simulink model "fft_overlap_tomori"  (R2023b)
settings: Solver=VariableStepAuto  StartTime=0.0  StopTime=inf  RelTol=1e-3
InitFcn:
  | fftparrallelout
  | load('dataram.mat')
  | s= fi(exp(-1j*2*pi.*(0:63)/64),1,16,15);
  | fixed_point = fixdt(1,27,20);
  | fixed_pointu = fixdt(0,29,20);
  | fixed = fixdt(1,22,15);
  | const = fixdt(1,18,17);
  | addConst = fixdt(1,18,16);
  | f =10.4e6;
  | f1=45e6;
  | alpha1 =5;
  | beta1 = 0.00001 ;
  | beta2 = 0.99999 ;
  | beta3 = 23;
undefined symbols (not defined in the file or in its folder): j
libraries: dspxfrm3 x11, commrflib2 x4
(part 5 of 10)

== system fft_overlap_tomori/FFT64_outMuxed/64pointFFTchan/FFT64/complexmult23 ==
  x1 : Inport
  In3 : Inport  Port=2
  Add1 : Sum  OutDataTypeStr=addConst  RndMeth=Round
  Add2 : Sum  Inputs=+-  OutDataTypeStr=fixed  AccumDataTypeStr=fixed  RndMeth=Round
  Add20 : Sum  OutDataTypeStr=fixed  RndMeth=Round
  Add3 : Sum  Inputs=+-  OutDataTypeStr=fixed  AccumDataTypeStr=fixed  RndMeth=Round
  Add4 : Sum  Inputs=+-  OutDataTypeStr=fixed  AccumDataTypeStr=fixed  RndMeth=Round
  Complex to Real-Imag : ComplexToRealImag
  Complex to Real-Imag1 : ComplexToRealImag
  Constant : Constant  Commented=on  Value=1+j  OutDataTypeStr=fixdt(1,22, 15)  SampleTime=2e-8
  Constant1 : Constant  Commented=on  Value=1-j  OutDataTypeStr=fixdt(1,22, 15)  SampleTime=2e-8
  Data Type Conversion : DataTypeConversion  OutDataTypeStr=fixed  RndMeth=Round  SaturateOnIntegerOverflow=off
  Data Type Conversion1 : DataTypeConversion  OutDataTypeStr=fixed  RndMeth=Round  SaturateOnIntegerOverflow=off
  Data Type Conversion2 : DataTypeConversion  OutDataTypeStr=fixed  RndMeth=Round  SaturateOnIntegerOverflow=off
  Delay : Delay
  Delay1 : Delay
  Delay{3..14} (12 alike) : Delay  DelayLength=1
  Delay2 : Delay
  Display : Display  Commented=on
  Product : Product
  Product1 : Product
  Product2 : Product
  Real-Imag to Complex : RealImagToComplex
  Out1 : Outport
  wires:
  Delay14/1 -> Add4/2, Delay11/1
  Data Type Conversion2/1 -> Delay14/1
  Delay13/1 -> Add3/2, Add4/1
  Data Type Conversion1/1 -> Delay13/1
  Data Type Conversion/1 -> Delay12/1
  Delay12/1 -> Add3/1
  Add2/1 -> Real-Imag to Complex/2
  Delay11/1 -> Add2/2
  Delay10/1 -> Add2/1
  Delay9/1 -> Real-Imag to Complex/1
  Delay8/1 -> Product2/2
  Delay7/1 -> Product2/1
  Delay6/1 -> Product1/2
  Delay5/1 -> Product1/1
  Delay4/1 -> Product/2
  Delay3/1 -> Product/1
  Complex to Real-Imag1/2 -> Add1/2, Delay8/1
  Complex to Real-Imag/2 -> Add20/2, Delay7/1
  Complex to Real-Imag1/1 -> Add1/1, Delay6/1
  Complex to Real-Imag/1 -> Add20/1, Delay5/1
  Add1/1 -> Delay4/1
  Add20/1 -> Delay3/1
  Add3/1 -> Delay10/1
  Add4/1 -> Delay9/1
  Delay2/1 -> Data Type Conversion2/1
  Delay1/1 -> Data Type Conversion1/1
  Delay/1 -> Data Type Conversion/1
  Product2/1 -> Delay2/1
  Product1/1 -> Delay1/1
  Product/1 -> Delay/1
  x1/1 -> Complex to Real-Imag/1
  In3/1 -> Complex to Real-Imag1/1
  Real-Imag to Complex/1 -> Out1/1

== system fft_overlap_tomori/FFT64_outMuxed/64pointFFTchan/FFT64/complexmult24 ==
  x1 : Inport
  In3 : Inport  Port=2
  Add1 : Sum  OutDataTypeStr=addConst  RndMeth=Round
  Add2 : Sum  Inputs=+-  OutDataTypeStr=fixed  AccumDataTypeStr=fixed  RndMeth=Round
  Add20 : Sum  OutDataTypeStr=fixed  RndMeth=Round
  Add3 : Sum  Inputs=+-  OutDataTypeStr=fixed  AccumDataTypeStr=fixed  RndMeth=Round
  Add4 : Sum  Inputs=+-  OutDataTypeStr=fixed  AccumDataTypeStr=fixed  RndMeth=Round
  Complex to Real-Imag : ComplexToRealImag
  Complex to Real-Imag1 : ComplexToRealImag
  Constant : Constant  Commented=on  Value=1+j  OutDataTypeStr=fixdt(1,22, 15)  SampleTime=2e-8
  Constant1 : Constant  Commented=on  Value=1-j  OutDataTypeStr=fixdt(1,22, 15)  SampleTime=2e-8
  Data Type Conversion : DataTypeConversion  OutDataTypeStr=fixed  RndMeth=Round  SaturateOnIntegerOverflow=off
  Data Type Conversion1 : DataTypeConversion  OutDataTypeStr=fixed  RndMeth=Round  SaturateOnIntegerOverflow=off
  Data Type Conversion2 : DataTypeConversion  OutDataTypeStr=fixed  RndMeth=Round  SaturateOnIntegerOverflow=off
  Delay : Delay
  Delay1 : Delay
  Delay{3..14} (12 alike) : Delay  DelayLength=1
  Delay2 : Delay
  Display : Display  Commented=on
  Product : Product
  Product1 : Product
  Product2 : Product
  Real-Imag to Complex : RealImagToComplex
  Out1 : Outport
  wires:
  Real-Imag to Complex/1 -> Out1/1
  In3/1 -> Complex to Real-Imag1/1
  x1/1 -> Complex to Real-Imag/1
  Product/1 -> Delay/1
  Product1/1 -> Delay1/1
  Product2/1 -> Delay2/1
  Delay/1 -> Data Type Conversion/1
  Delay1/1 -> Data Type Conversion1/1
  Delay2/1 -> Data Type Conversion2/1
  Add4/1 -> Delay9/1
  Add3/1 -> Delay10/1
  Add20/1 -> Delay3/1
  Add1/1 -> Delay4/1
  Complex to Real-Imag/1 -> Delay5/1, Add20/1
  Complex to Real-Imag1/1 -> Delay6/1, Add1/1
  Complex to Real-Imag/2 -> Delay7/1, Add20/2
  Complex to Real-Imag1/2 -> Delay8/1, Add1/2
  Delay3/1 -> Product/1
  Delay4/1 -> Product/2
  Delay5/1 -> Product1/1
  Delay6/1 -> Product1/2
  Delay7/1 -> Product2/1
  Delay8/1 -> Product2/2
  Delay9/1 -> Real-Imag to Complex/1
  Delay10/1 -> Add2/1
  Delay11/1 -> Add2/2
  Add2/1 -> Real-Imag to Complex/2
  Delay12/1 -> Add3/1
  Data Type Conversion/1 -> Delay12/1
  Data Type Conversion1/1 -> Delay13/1
  Delay13/1 -> Add4/1, Add3/2
  Data Type Conversion2/1 -> Delay14/1
  Delay14/1 -> Delay11/1, Add4/2

== system fft_overlap_tomori/FFT64_outMuxed/64pointFFTchan/FFT64/complexmult25 ==
  x1 : Inport
  In3 : Inport  Port=2
  Add1 : Sum  OutDataTypeStr=addConst  RndMeth=Round
  Add2 : Sum  Inputs=+-  OutDataTypeStr=fixed  AccumDataTypeStr=fixed  RndMeth=Round
  Add20 : Sum  OutDataTypeStr=fixed  RndMeth=Round
  Add3 : Sum  Inputs=+-  OutDataTypeStr=fixed  AccumDataTypeStr=fixed  RndMeth=Round
  Add4 : Sum  Inputs=+-  OutDataTypeStr=fixed  AccumDataTypeStr=fixed  RndMeth=Round
  Complex to Real-Imag : ComplexToRealImag
  Complex to Real-Imag1 : ComplexToRealImag
  Constant : Constant  Commented=on  Value=1+j  OutDataTypeStr=fixdt(1,22, 15)  SampleTime=2e-8
  Constant1 : Constant  Commented=on  Value=1-j  OutDataTypeStr=fixdt(1,22, 15)  SampleTime=2e-8
  Data Type Conversion : DataTypeConversion  OutDataTypeStr=fixed  RndMeth=Round  SaturateOnIntegerOverflow=off
  Data Type Conversion1 : DataTypeConversion  OutDataTypeStr=fixed  RndMeth=Round  SaturateOnIntegerOverflow=off
  Data Type Conversion2 : DataTypeConversion  OutDataTypeStr=fixed  RndMeth=Round  SaturateOnIntegerOverflow=off
  Delay : Delay
  Delay1 : Delay
  Delay{3..14} (12 alike) : Delay  DelayLength=1
  Delay2 : Delay
  Display : Display  Commented=on
  Product : Product
  Product1 : Product
  Product2 : Product
  Real-Imag to Complex : RealImagToComplex
  Out1 : Outport
  wires:
  Delay14/1 -> Add4/2, Delay11/1
  Data Type Conversion2/1 -> Delay14/1
  Delay13/1 -> Add3/2, Add4/1
  Data Type Conversion1/1 -> Delay13/1
  Data Type Conversion/1 -> Delay12/1
  Delay12/1 -> Add3/1
  Add2/1 -> Real-Imag to Complex/2
  Delay11/1 -> Add2/2
  Delay10/1 -> Add2/1
  Delay9/1 -> Real-Imag to Complex/1
  Delay8/1 -> Product2/2
  Delay7/1 -> Product2/1
  Delay6/1 -> Product1/2
  Delay5/1 -> Product1/1
  Delay4/1 -> Product/2
  Delay3/1 -> Product/1
  Complex to Real-Imag1/2 -> Add1/2, Delay8/1
  Complex to Real-Imag/2 -> Add20/2, Delay7/1
  Complex to Real-Imag1/1 -> Add1/1, Delay6/1
  Complex to Real-Imag/1 -> Add20/1, Delay5/1
  Add1/1 -> Delay4/1
  Add20/1 -> Delay3/1
  Add3/1 -> Delay10/1
  Add4/1 -> Delay9/1
  Delay2/1 -> Data Type Conversion2/1
  Delay1/1 -> Data Type Conversion1/1
  Delay/1 -> Data Type Conversion/1
  Product2/1 -> Delay2/1
  Product1/1 -> Delay1/1
  Product/1 -> Delay/1
  x1/1 -> Complex to Real-Imag/1
  In3/1 -> Complex to Real-Imag1/1
  Real-Imag to Complex/1 -> Out1/1

== system fft_overlap_tomori/FFT64_outMuxed/64pointFFTchan/FFT64/complexmult26 ==
  x1 : Inport
  In3 : Inport  Port=2
  Add1 : Sum  OutDataTypeStr=addConst  RndMeth=Round
  Add2 : Sum  Inputs=+-  OutDataTypeStr=fixed  AccumDataTypeStr=fixed  RndMeth=Round
  Add20 : Sum  OutDataTypeStr=fixed  RndMeth=Round
  Add3 : Sum  Inputs=+-  OutDataTypeStr=fixed  AccumDataTypeStr=fixed  RndMeth=Round
  Add4 : Sum  Inputs=+-  OutDataTypeStr=fixed  AccumDataTypeStr=fixed  RndMeth=Round
  Complex to Real-Imag : ComplexToRealImag
  Complex to Real-Imag1 : ComplexToRealImag
  Constant : Constant  Commented=on  Value=1+j  OutDataTypeStr=fixdt(1,22, 15)  SampleTime=2e-8
  Constant1 : Constant  Commented=on  Value=1-j  OutDataTypeStr=fixdt(1,22, 15)  SampleTime=2e-8
  Data Type Conversion : DataTypeConversion  OutDataTypeStr=fixed  RndMeth=Round  SaturateOnIntegerOverflow=off
  Data Type Conversion1 : DataTypeConversion  OutDataTypeStr=fixed  RndMeth=Round  SaturateOnIntegerOverflow=off
  Data Type Conversion2 : DataTypeConversion  OutDataTypeStr=fixed  RndMeth=Round  SaturateOnIntegerOverflow=off
  Delay : Delay
  Delay1 : Delay
  Delay{3..14} (12 alike) : Delay  DelayLength=1
  Delay2 : Delay
  Display : Display  Commented=on
  Product : Product
  Product1 : Product
  Product2 : Product
  Real-Imag to Complex : RealImagToComplex
  Out1 : Outport
  wires:
  Real-Imag to Complex/1 -> Out1/1
  In3/1 -> Complex to Real-Imag1/1
  x1/1 -> Complex to Real-Imag/1
  Product/1 -> Delay/1
  Product1/1 -> Delay1/1
  Product2/1 -> Delay2/1
  Delay/1 -> Data Type Conversion/1
  Delay1/1 -> Data Type Conversion1/1
  Delay2/1 -> Data Type Conversion2/1
  Add4/1 -> Delay9/1
  Add3/1 -> Delay10/1
  Add20/1 -> Delay3/1
  Add1/1 -> Delay4/1
  Complex to Real-Imag/1 -> Delay5/1, Add20/1
  Complex to Real-Imag1/1 -> Delay6/1, Add1/1
  Complex to Real-Imag/2 -> Delay7/1, Add20/2
  Complex to Real-Imag1/2 -> Delay8/1, Add1/2
  Delay3/1 -> Product/1
  Delay4/1 -> Product/2
  Delay5/1 -> Product1/1
  Delay6/1 -> Product1/2
  Delay7/1 -> Product2/1
  Delay8/1 -> Product2/2
  Delay9/1 -> Real-Imag to Complex/1
  Delay10/1 -> Add2/1
  Delay11/1 -> Add2/2
  Add2/1 -> Real-Imag to Complex/2
  Delay12/1 -> Add3/1
  Data Type Conversion/1 -> Delay12/1
  Data Type Conversion1/1 -> Delay13/1
  Delay13/1 -> Add4/1, Add3/2
  Data Type Conversion2/1 -> Delay14/1
  Delay14/1 -> Delay11/1, Add4/2

== system fft_overlap_tomori/FFT64_outMuxed/64pointFFTchan/FFT64/complexmult27 ==
  x1 : Inport
  In3 : Inport  Port=2
  Add1 : Sum  OutDataTypeStr=addConst  RndMeth=Round
  Add2 : Sum  Inputs=+-  OutDataTypeStr=fixed  AccumDataTypeStr=fixed  RndMeth=Round
  Add20 : Sum  OutDataTypeStr=fixed  RndMeth=Round
  Add3 : Sum  Inputs=+-  OutDataTypeStr=fixed  AccumDataTypeStr=fixed  RndMeth=Round
  Add4 : Sum  Inputs=+-  OutDataTypeStr=fixed  AccumDataTypeStr=fixed  RndMeth=Round
  Complex to Real-Imag : ComplexToRealImag
  Complex to Real-Imag1 : ComplexToRealImag
  Constant : Constant  Commented=on  Value=1+j  OutDataTypeStr=fixdt(1,22, 15)  SampleTime=2e-8
  Constant1 : Constant  Commented=on  Value=1-j  OutDataTypeStr=fixdt(1,22, 15)  SampleTime=2e-8
  Data Type Conversion : DataTypeConversion  OutDataTypeStr=fixed  RndMeth=Round  SaturateOnIntegerOverflow=off
  Data Type Conversion1 : DataTypeConversion  OutDataTypeStr=fixed  RndMeth=Round  SaturateOnIntegerOverflow=off
  Data Type Conversion2 : DataTypeConversion  OutDataTypeStr=fixed  RndMeth=Round  SaturateOnIntegerOverflow=off
  Delay : Delay
  Delay1 : Delay
  Delay{3..14} (12 alike) : Delay  DelayLength=1
  Delay2 : Delay
  Display : Display  Commented=on
  Product : Product
  Product1 : Product
  Product2 : Product
  Real-Imag to Complex : RealImagToComplex
  Out1 : Outport
  wires:
  Delay14/1 -> Add4/2, Delay11/1
  Data Type Conversion2/1 -> Delay14/1
  Delay13/1 -> Add3/2, Add4/1
  Data Type Conversion1/1 -> Delay13/1
  Data Type Conversion/1 -> Delay12/1
  Delay12/1 -> Add3/1
  Add2/1 -> Real-Imag to Complex/2
  Delay11/1 -> Add2/2
  Delay10/1 -> Add2/1
  Delay9/1 -> Real-Imag to Complex/1
  Delay8/1 -> Product2/2
  Delay7/1 -> Product2/1
  Delay6/1 -> Product1/2
  Delay5/1 -> Product1/1
  Delay4/1 -> Product/2
  Delay3/1 -> Product/1
  Complex to Real-Imag1/2 -> Add1/2, Delay8/1
  Complex to Real-Imag/2 -> Add20/2, Delay7/1
  Complex to Real-Imag1/1 -> Add1/1, Delay6/1
  Complex to Real-Imag/1 -> Add20/1, Delay5/1
  Add1/1 -> Delay4/1
  Add20/1 -> Delay3/1
  Add3/1 -> Delay10/1
  Add4/1 -> Delay9/1
  Delay2/1 -> Data Type Conversion2/1
  Delay1/1 -> Data Type Conversion1/1
  Delay/1 -> Data Type Conversion/1
  Product2/1 -> Delay2/1
  Product1/1 -> Delay1/1
  Product/1 -> Delay/1
  x1/1 -> Complex to Real-Imag/1
  In3/1 -> Complex to Real-Imag1/1
  Real-Imag to Complex/1 -> Out1/1

== system fft_overlap_tomori/FFT64_outMuxed/64pointFFTchan/FFT64/complexmult3 ==
  x1 : Inport
  In3 : Inport  Port=2
  Add1 : Sum  OutDataTypeStr=addConst  RndMeth=Round
  Add2 : Sum  Inputs=+-  OutDataTypeStr=fixed  AccumDataTypeStr=fixed  RndMeth=Round
  Add20 : Sum  OutDataTypeStr=fixed  RndMeth=Round
  Add3 : Sum  Inputs=+-  OutDataTypeStr=fixed  AccumDataTypeStr=fixed  RndMeth=Round
  Add4 : Sum  Inputs=+-  OutDataTypeStr=fixed  AccumDataTypeStr=fixed  RndMeth=Round
  Complex to Real-Imag : ComplexToRealImag
  Complex to Real-Imag1 : ComplexToRealImag
  Constant : Constant  Commented=on  Value=1+j  OutDataTypeStr=fixdt(1,22, 15)  SampleTime=2e-8
  Constant1 : Constant  Commented=on  Value=1-j  OutDataTypeStr=fixdt(1,22, 15)  SampleTime=2e-8
  Data Type Conversion : DataTypeConversion  OutDataTypeStr=fixed  RndMeth=Round  SaturateOnIntegerOverflow=off
  Data Type Conversion1 : DataTypeConversion  OutDataTypeStr=fixed  RndMeth=Round  SaturateOnIntegerOverflow=off
  Data Type Conversion2 : DataTypeConversion  OutDataTypeStr=fixed  RndMeth=Round  SaturateOnIntegerOverflow=off
  Delay : Delay
  Delay1 : Delay
  Delay{3..14} (12 alike) : Delay  DelayLength=1
  Delay2 : Delay
  Display : Display  Commented=on
  Product : Product
  Product1 : Product
  Product2 : Product
  Real-Imag to Complex : RealImagToComplex
  Out1 : Outport
  wires:
  Delay14/1 -> Add4/2, Delay11/1
  Data Type Conversion2/1 -> Delay14/1
  Delay13/1 -> Add3/2, Add4/1
  Data Type Conversion1/1 -> Delay13/1
  Data Type Conversion/1 -> Delay12/1
  Delay12/1 -> Add3/1
  Add2/1 -> Real-Imag to Complex/2
  Delay11/1 -> Add2/2
  Delay10/1 -> Add2/1
  Delay9/1 -> Real-Imag to Complex/1
  Delay8/1 -> Product2/2
  Delay7/1 -> Product2/1
  Delay6/1 -> Product1/2
  Delay5/1 -> Product1/1
  Delay4/1 -> Product/2
  Delay3/1 -> Product/1
  Complex to Real-Imag1/2 -> Add1/2, Delay8/1
  Complex to Real-Imag/2 -> Add20/2, Delay7/1
  Complex to Real-Imag1/1 -> Add1/1, Delay6/1
  Complex to Real-Imag/1 -> Add20/1, Delay5/1
  Add1/1 -> Delay4/1
  Add20/1 -> Delay3/1
  Add3/1 -> Delay10/1
  Add4/1 -> Delay9/1
  Delay2/1 -> Data Type Conversion2/1
  Delay1/1 -> Data Type Conversion1/1
  Delay/1 -> Data Type Conversion/1
  Product2/1 -> Delay2/1
  Product1/1 -> Delay1/1
  Product/1 -> Delay/1
  x1/1 -> Complex to Real-Imag/1
  In3/1 -> Complex to Real-Imag1/1
  Real-Imag to Complex/1 -> Out1/1

== system fft_overlap_tomori/FFT64_outMuxed/64pointFFTchan/FFT64/complexmult4 ==
  x1 : Inport
  In3 : Inport  Port=2
  Add1 : Sum  OutDataTypeStr=addConst  RndMeth=Round
  Add2 : Sum  Inputs=+-  OutDataTypeStr=fixed  AccumDataTypeStr=fixed  RndMeth=Round
  Add20 : Sum  OutDataTypeStr=fixed  RndMeth=Round
  Add3 : Sum  Inputs=+-  OutDataTypeStr=fixed  AccumDataTypeStr=fixed  RndMeth=Round
  Add4 : Sum  Inputs=+-  OutDataTypeStr=fixed  AccumDataTypeStr=fixed  RndMeth=Round
  Complex to Real-Imag : ComplexToRealImag
  Complex to Real-Imag1 : ComplexToRealImag
  Constant : Constant  Commented=on  Value=1+j  OutDataTypeStr=fixdt(1,22, 15)  SampleTime=2e-8
  Constant1 : Constant  Commented=on  Value=1-j  OutDataTypeStr=fixdt(1,22, 15)  SampleTime=2e-8
  Data Type Conversion : DataTypeConversion  OutDataTypeStr=fixed  RndMeth=Round  SaturateOnIntegerOverflow=off
  Data Type Conversion1 : DataTypeConversion  OutDataTypeStr=fixed  RndMeth=Round  SaturateOnIntegerOverflow=off
  Data Type Conversion2 : DataTypeConversion  OutDataTypeStr=fixed  RndMeth=Round  SaturateOnIntegerOverflow=off
  Delay : Delay
  Delay1 : Delay
  Delay{3..14} (12 alike) : Delay  DelayLength=1
  Delay2 : Delay
  Display : Display  Commented=on
  Product : Product
  Product1 : Product
  Product2 : Product
  Real-Imag to Complex : RealImagToComplex
  Out1 : Outport
  wires:
  Real-Imag to Complex/1 -> Out1/1
  In3/1 -> Complex to Real-Imag1/1
  x1/1 -> Complex to Real-Imag/1
  Product/1 -> Delay/1
  Product1/1 -> Delay1/1
  Product2/1 -> Delay2/1
  Delay/1 -> Data Type Conversion/1
  Delay1/1 -> Data Type Conversion1/1
  Delay2/1 -> Data Type Conversion2/1
  Add4/1 -> Delay9/1
  Add3/1 -> Delay10/1
  Add20/1 -> Delay3/1
  Add1/1 -> Delay4/1
  Complex to Real-Imag/1 -> Delay5/1, Add20/1
  Complex to Real-Imag1/1 -> Delay6/1, Add1/1
  Complex to Real-Imag/2 -> Delay7/1, Add20/2
  Complex to Real-Imag1/2 -> Delay8/1, Add1/2
  Delay3/1 -> Product/1
  Delay4/1 -> Product/2
  Delay5/1 -> Product1/1
  Delay6/1 -> Product1/2
  Delay7/1 -> Product2/1
  Delay8/1 -> Product2/2
  Delay9/1 -> Real-Imag to Complex/1
  Delay10/1 -> Add2/1
  Delay11/1 -> Add2/2
  Add2/1 -> Real-Imag to Complex/2
  Delay12/1 -> Add3/1
  Data Type Conversion/1 -> Delay12/1
  Data Type Conversion1/1 -> Delay13/1
  Delay13/1 -> Add4/1, Add3/2
  Data Type Conversion2/1 -> Delay14/1
  Delay14/1 -> Delay11/1, Add4/2

== system fft_overlap_tomori/FFT64_outMuxed/64pointFFTchan/FFT64/complexmult5 ==
  x1 : Inport
  In3 : Inport  Port=2
  Add1 : Sum  OutDataTypeStr=addConst  RndMeth=Round
  Add2 : Sum  Inputs=+-  OutDataTypeStr=fixed  AccumDataTypeStr=fixed  RndMeth=Round
  Add20 : Sum  OutDataTypeStr=fixed  RndMeth=Round
  Add3 : Sum  Inputs=+-  OutDataTypeStr=fixed  AccumDataTypeStr=fixed  RndMeth=Round
  Add4 : Sum  Inputs=+-  OutDataTypeStr=fixed  AccumDataTypeStr=fixed  RndMeth=Round
  Complex to Real-Imag : ComplexToRealImag
  Complex to Real-Imag1 : ComplexToRealImag
  Constant : Constant  Commented=on  Value=1+j  OutDataTypeStr=fixdt(1,22, 15)  SampleTime=2e-8
  Constant1 : Constant  Commented=on  Value=1-j  OutDataTypeStr=fixdt(1,22, 15)  SampleTime=2e-8
  Data Type Conversion : DataTypeConversion  OutDataTypeStr=fixed  RndMeth=Round  SaturateOnIntegerOverflow=off
  Data Type Conversion1 : DataTypeConversion  OutDataTypeStr=fixed  RndMeth=Round  SaturateOnIntegerOverflow=off
  Data Type Conversion2 : DataTypeConversion  OutDataTypeStr=fixed  RndMeth=Round  SaturateOnIntegerOverflow=off
  Delay : Delay
  Delay1 : Delay
  Delay{3..14} (12 alike) : Delay  DelayLength=1
  Delay2 : Delay
  Display : Display  Commented=on
  Product : Product
  Product1 : Product
  Product2 : Product
  Real-Imag to Complex : RealImagToComplex
  Out1 : Outport
  wires:
  Delay14/1 -> Add4/2, Delay11/1
  Data Type Conversion2/1 -> Delay14/1
  Delay13/1 -> Add3/2, Add4/1
  Data Type Conversion1/1 -> Delay13/1
  Data Type Conversion/1 -> Delay12/1
  Delay12/1 -> Add3/1
  Add2/1 -> Real-Imag to Complex/2
  Delay11/1 -> Add2/2
  Delay10/1 -> Add2/1
  Delay9/1 -> Real-Imag to Complex/1
  Delay8/1 -> Product2/2
  Delay7/1 -> Product2/1
  Delay6/1 -> Product1/2
  Delay5/1 -> Product1/1
  Delay4/1 -> Product/2
  Delay3/1 -> Product/1
  Complex to Real-Imag1/2 -> Add1/2, Delay8/1
  Complex to Real-Imag/2 -> Add20/2, Delay7/1
  Complex to Real-Imag1/1 -> Add1/1, Delay6/1
  Complex to Real-Imag/1 -> Add20/1, Delay5/1
  Add1/1 -> Delay4/1
  Add20/1 -> Delay3/1
  Add3/1 -> Delay10/1
  Add4/1 -> Delay9/1
  Delay2/1 -> Data Type Conversion2/1
  Delay1/1 -> Data Type Conversion1/1
  Delay/1 -> Data Type Conversion/1
  Product2/1 -> Delay2/1
  Product1/1 -> Delay1/1
  Product/1 -> Delay/1
  x1/1 -> Complex to Real-Imag/1
  In3/1 -> Complex to Real-Imag1/1
  Real-Imag to Complex/1 -> Out1/1

== system fft_overlap_tomori/FFT64_outMuxed/64pointFFTchan/FFT64/complexmult6 ==
  x1 : Inport
  In3 : Inport  Port=2
  Add1 : Sum  OutDataTypeStr=addConst  RndMeth=Round
  Add2 : Sum  Inputs=+-  OutDataTypeStr=fixed  AccumDataTypeStr=fixed  RndMeth=Round
  Add20 : Sum  OutDataTypeStr=fixed  RndMeth=Round
  Add3 : Sum  Inputs=+-  OutDataTypeStr=fixed  AccumDataTypeStr=fixed  RndMeth=Round
  Add4 : Sum  Inputs=+-  OutDataTypeStr=fixed  AccumDataTypeStr=fixed  RndMeth=Round
  Complex to Real-Imag : ComplexToRealImag
  Complex to Real-Imag1 : ComplexToRealImag
  Constant : Constant  Commented=on  Value=1+j  OutDataTypeStr=fixdt(1,22, 15)  SampleTime=2e-8
  Constant1 : Constant  Commented=on  Value=1-j  OutDataTypeStr=fixdt(1,22, 15)  SampleTime=2e-8
  Data Type Conversion : DataTypeConversion  OutDataTypeStr=fixed  RndMeth=Round  SaturateOnIntegerOverflow=off
  Data Type Conversion1 : DataTypeConversion  OutDataTypeStr=fixed  RndMeth=Round  SaturateOnIntegerOverflow=off
  Data Type Conversion2 : DataTypeConversion  OutDataTypeStr=fixed  RndMeth=Round  SaturateOnIntegerOverflow=off
  Delay : Delay
  Delay1 : Delay
  Delay{3..14} (12 alike) : Delay  DelayLength=1
  Delay2 : Delay
  Display : Display  Commented=on
  Product : Product
  Product1 : Product
  Product2 : Product
  Real-Imag to Complex : RealImagToComplex
  Out1 : Outport
  wires:
  Real-Imag to Complex/1 -> Out1/1
  In3/1 -> Complex to Real-Imag1/1
  x1/1 -> Complex to Real-Imag/1
  Product/1 -> Delay/1
  Product1/1 -> Delay1/1
  Product2/1 -> Delay2/1
  Delay/1 -> Data Type Conversion/1
  Delay1/1 -> Data Type Conversion1/1
  Delay2/1 -> Data Type Conversion2/1
  Add4/1 -> Delay9/1
  Add3/1 -> Delay10/1
  Add20/1 -> Delay3/1
  Add1/1 -> Delay4/1
  Complex to Real-Imag/1 -> Delay5/1, Add20/1
  Complex to Real-Imag1/1 -> Delay6/1, Add1/1
  Complex to Real-Imag/2 -> Delay7/1, Add20/2
  Complex to Real-Imag1/2 -> Delay8/1, Add1/2
  Delay3/1 -> Product/1
  Delay4/1 -> Product/2
  Delay5/1 -> Product1/1
  Delay6/1 -> Product1/2
  Delay7/1 -> Product2/1
  Delay8/1 -> Product2/2
  Delay9/1 -> Real-Imag to Complex/1
  Delay10/1 -> Add2/1
  Delay11/1 -> Add2/2
  Add2/1 -> Real-Imag to Complex/2
  Delay12/1 -> Add3/1
  Data Type Conversion/1 -> Delay12/1
  Data Type Conversion1/1 -> Delay13/1
  Delay13/1 -> Add4/1, Add3/2
  Data Type Conversion2/1 -> Delay14/1
  Delay14/1 -> Delay11/1, Add4/2

== system fft_overlap_tomori/FFT64_outMuxed/64pointFFTchan/FFT64/complexmult7 ==
  x1 : Inport
  In3 : Inport  Port=2
  Add1 : Sum  OutDataTypeStr=addConst  RndMeth=Round
  Add2 : Sum  Inputs=+-  OutDataTypeStr=fixed  AccumDataTypeStr=fixed  RndMeth=Round
  Add20 : Sum  OutDataTypeStr=fixed  RndMeth=Round
  Add3 : Sum  Inputs=+-  OutDataTypeStr=fixed  AccumDataTypeStr=fixed  RndMeth=Round
  Add4 : Sum  Inputs=+-  OutDataTypeStr=fixed  AccumDataTypeStr=fixed  RndMeth=Round
  Complex to Real-Imag : ComplexToRealImag
  Complex to Real-Imag1 : ComplexToRealImag
  Constant : Constant  Commented=on  Value=1+j  OutDataTypeStr=fixdt(1,22, 15)  SampleTime=2e-8
  Constant1 : Constant  Commented=on  Value=1-j  OutDataTypeStr=fixdt(1,22, 15)  SampleTime=2e-8
  Data Type Conversion : DataTypeConversion  OutDataTypeStr=fixed  RndMeth=Round  SaturateOnIntegerOverflow=off
  Data Type Conversion1 : DataTypeConversion  OutDataTypeStr=fixed  RndMeth=Round  SaturateOnIntegerOverflow=off
  Data Type Conversion2 : DataTypeConversion  OutDataTypeStr=fixed  RndMeth=Round  SaturateOnIntegerOverflow=off
  Delay : Delay
  Delay1 : Delay
  Delay{3..14} (12 alike) : Delay  DelayLength=1
  Delay2 : Delay
  Display : Display  Commented=on
  Product : Product
  Product1 : Product
  Product2 : Product
  Real-Imag to Complex : RealImagToComplex
  Out1 : Outport
  wires:
  Delay14/1 -> Add4/2, Delay11/1
  Data Type Conversion2/1 -> Delay14/1
  Delay13/1 -> Add3/2, Add4/1
  Data Type Conversion1/1 -> Delay13/1
  Data Type Conversion/1 -> Delay12/1
  Delay12/1 -> Add3/1
  Add2/1 -> Real-Imag to Complex/2
  Delay11/1 -> Add2/2
  Delay10/1 -> Add2/1
  Delay9/1 -> Real-Imag to Complex/1
  Delay8/1 -> Product2/2
  Delay7/1 -> Product2/1
  Delay6/1 -> Product1/2
  Delay5/1 -> Product1/1
  Delay4/1 -> Product/2
  Delay3/1 -> Product/1
  Complex to Real-Imag1/2 -> Add1/2, Delay8/1
  Complex to Real-Imag/2 -> Add20/2, Delay7/1
  Complex to Real-Imag1/1 -> Add1/1, Delay6/1
  Complex to Real-Imag/1 -> Add20/1, Delay5/1
  Add1/1 -> Delay4/1
  Add20/1 -> Delay3/1
  Add3/1 -> Delay10/1
  Add4/1 -> Delay9/1
  Delay2/1 -> Data Type Conversion2/1
  Delay1/1 -> Data Type Conversion1/1
  Delay/1 -> Data Type Conversion/1
  Product2/1 -> Delay2/1
  Product1/1 -> Delay1/1
  Product/1 -> Delay/1
  x1/1 -> Complex to Real-Imag/1
  In3/1 -> Complex to Real-Imag1/1
  Real-Imag to Complex/1 -> Out1/1

== system fft_overlap_tomori/FFT64_outMuxed/64pointFFTchan/FFT64/complexmult8 ==
  x1 : Inport
  In3 : Inport  Port=2
  Add1 : Sum  OutDataTypeStr=addConst  RndMeth=Round
  Add2 : Sum  Inputs=+-  OutDataTypeStr=fixed  AccumDataTypeStr=fixed  RndMeth=Round
  Add20 : Sum  OutDataTypeStr=fixed  RndMeth=Round
  Add3 : Sum  Inputs=+-  OutDataTypeStr=fixed  AccumDataTypeStr=fixed  RndMeth=Round
  Add4 : Sum  Inputs=+-  OutDataTypeStr=fixed  AccumDataTypeStr=fixed  RndMeth=Round
  Complex to Real-Imag : ComplexToRealImag
  Complex to Real-Imag1 : ComplexToRealImag
  Constant : Constant  Commented=on  Value=1+j  OutDataTypeStr=fixdt(1,22, 15)  SampleTime=2e-8
  Constant1 : Constant  Commented=on  Value=1-j  OutDataTypeStr=fixdt(1,22, 15)  SampleTime=2e-8
  Data Type Conversion : DataTypeConversion  OutDataTypeStr=fixed  RndMeth=Round  SaturateOnIntegerOverflow=off
  Data Type Conversion1 : DataTypeConversion  OutDataTypeStr=fixed  RndMeth=Round  SaturateOnIntegerOverflow=off
  Data Type Conversion2 : DataTypeConversion  OutDataTypeStr=fixed  RndMeth=Round  SaturateOnIntegerOverflow=off
  Delay : Delay
  Delay1 : Delay
  Delay{3..14} (12 alike) : Delay  DelayLength=1
  Delay2 : Delay
  Display : Display  Commented=on
  Product : Product
  Product1 : Product
  Product2 : Product
  Real-Imag to Complex : RealImagToComplex
  Out1 : Outport
  wires:
  Real-Imag to Complex/1 -> Out1/1
  In3/1 -> Complex to Real-Imag1/1
  x1/1 -> Complex to Real-Imag/1
  Product/1 -> Delay/1
  Product1/1 -> Delay1/1
  Product2/1 -> Delay2/1
  Delay/1 -> Data Type Conversion/1
  Delay1/1 -> Data Type Conversion1/1
  Delay2/1 -> Data Type Conversion2/1
  Add4/1 -> Delay9/1
  Add3/1 -> Delay10/1
  Add20/1 -> Delay3/1
  Add1/1 -> Delay4/1
  Complex to Real-Imag/1 -> Delay5/1, Add20/1
  Complex to Real-Imag1/1 -> Delay6/1, Add1/1
  Complex to Real-Imag/2 -> Delay7/1, Add20/2
  Complex to Real-Imag1/2 -> Delay8/1, Add1/2
  Delay3/1 -> Product/1
  Delay4/1 -> Product/2
  Delay5/1 -> Product1/1
  Delay6/1 -> Product1/2
  Delay7/1 -> Product2/1
  Delay8/1 -> Product2/2
  Delay9/1 -> Real-Imag to Complex/1
  Delay10/1 -> Add2/1
  Delay11/1 -> Add2/2
  Add2/1 -> Real-Imag to Complex/2
  Delay12/1 -> Add3/1
  Data Type Conversion/1 -> Delay12/1
  Data Type Conversion1/1 -> Delay13/1
  Delay13/1 -> Add4/1, Add3/2
  Data Type Conversion2/1 -> Delay14/1
  Delay14/1 -> Delay11/1, Add4/2

== system fft_overlap_tomori/FFT64_outMuxed/64pointFFTchan/FFT64/complexmult9 ==
  x1 : Inport
  In3 : Inport  Port=2
  Add1 : Sum  OutDataTypeStr=addConst  RndMeth=Round
  Add2 : Sum  Inputs=+-  OutDataTypeStr=fixed  AccumDataTypeStr=fixed  RndMeth=Round
  Add20 : Sum  OutDataTypeStr=fixed  RndMeth=Round
  Add3 : Sum  Inputs=+-  OutDataTypeStr=fixed  AccumDataTypeStr=fixed  RndMeth=Round
  Add4 : Sum  Inputs=+-  OutDataTypeStr=fixed  AccumDataTypeStr=fixed  RndMeth=Round
  Complex to Real-Imag : ComplexToRealImag
  Complex to Real-Imag1 : ComplexToRealImag
  Constant : Constant  Commented=on  Value=1+j  OutDataTypeStr=fixdt(1,22, 15)  SampleTime=2e-8
  Constant1 : Constant  Commented=on  Value=1-j  OutDataTypeStr=fixdt(1,22, 15)  SampleTime=2e-8
  Data Type Conversion : DataTypeConversion  OutDataTypeStr=fixed  RndMeth=Round  SaturateOnIntegerOverflow=off
  Data Type Conversion1 : DataTypeConversion  OutDataTypeStr=fixed  RndMeth=Round  SaturateOnIntegerOverflow=off
  Data Type Conversion2 : DataTypeConversion  OutDataTypeStr=fixed  RndMeth=Round  SaturateOnIntegerOverflow=off
  Delay : Delay
  Delay1 : Delay
  Delay{3..14} (12 alike) : Delay  DelayLength=1
  Delay2 : Delay
  Display : Display  Commented=on
  Product : Product
  Product1 : Product
  Product2 : Product
  Real-Imag to Complex : RealImagToComplex
  Out1 : Outport
  wires:
  Delay14/1 -> Add4/2, Delay11/1
  Data Type Conversion2/1 -> Delay14/1
  Delay13/1 -> Add3/2, Add4/1
  Data Type Conversion1/1 -> Delay13/1
  Data Type Conversion/1 -> Delay12/1
  Delay12/1 -> Add3/1
  Add2/1 -> Real-Imag to Complex/2
  Delay11/1 -> Add2/2
  Delay10/1 -> Add2/1
  Delay9/1 -> Real-Imag to Complex/1
  Delay8/1 -> Product2/2
  Delay7/1 -> Product2/1
  Delay6/1 -> Product1/2
  Delay5/1 -> Product1/1
  Delay4/1 -> Product/2
  Delay3/1 -> Product/1
  Complex to Real-Imag1/2 -> Add1/2, Delay8/1
  Complex to Real-Imag/2 -> Add20/2, Delay7/1
  Complex to Real-Imag1/1 -> Add1/1, Delay6/1
  Complex to Real-Imag/1 -> Add20/1, Delay5/1
  Add1/1 -> Delay4/1
  Add20/1 -> Delay3/1
  Add3/1 -> Delay10/1
  Add4/1 -> Delay9/1
  Delay2/1 -> Data Type Conversion2/1
  Delay1/1 -> Data Type Conversion1/1
  Delay/1 -> Data Type Conversion/1
  Product2/1 -> Delay2/1
  Product1/1 -> Delay1/1
  Product/1 -> Delay/1
  x1/1 -> Complex to Real-Imag/1
  In3/1 -> Complex to Real-Imag1/1
  Real-Imag to Complex/1 -> Out1/1

== system fft_overlap_tomori/FFT64_outMuxed/64pointFFTchan/FFT64/multByExp(-j*Pi//4) ==
  x4 : Inport
  Add : Sum  OutDataTypeStr=fixed  RndMeth=Round
  Add1 : Sum  Inputs=+-  OutDataTypeStr=fixed  RndMeth=Round
  Complex to Real-Imag : ComplexToRealImag
  Data Type Conversion : DataTypeConversion  OutDataTypeStr=fixed  RndMeth=Round  SaturateOnIntegerOverflow=off
  Delay1 : Delay  DelayLength=1
  Delay24 : Delay  DelayLength=1
  Gain : Gain  Gain=sqrt(2)/2  ParamDataTypeStr=const
  Real-Imag to Complex : RealImagToComplex
  Out1 : Outport
  wires:
  x4/1 -> Gain/1
  Real-Imag to Complex/1 -> Out1/1
  Delay24/1 -> Complex to Real-Imag/1
  Add1/1 -> Real-Imag to Complex/2
  Add/1 -> Real-Imag to Complex/1
  Complex to Real-Imag/2 -> Add/2, Add1/1
  Complex to Real-Imag/1 -> Add/1, Add1/2
  Gain/1 -> Delay1/1
  Delay1/1 -> Data Type Conversion/1
  Data Type Conversion/1 -> Delay24/1

== system fft_overlap_tomori/FFT64_outMuxed/64pointFFTchan/FFT64/multByExp(-j*Pi//4)1 ==
  x4 : Inport
  Add : Sum  OutDataTypeStr=fixed  RndMeth=Round
  Add1 : Sum  Inputs=+-  OutDataTypeStr=fixed  RndMeth=Round
  Complex to Real-Imag : ComplexToRealImag
  Data Type Conversion : DataTypeConversion  OutDataTypeStr=fixed  RndMeth=Round  SaturateOnIntegerOverflow=off
  Delay1 : Delay  DelayLength=1
  Delay24 : Delay  DelayLength=1
  Gain : Gain  Gain=sqrt(2)/2  ParamDataTypeStr=const
  Real-Imag to Complex : RealImagToComplex
  Out1 : Outport
  wires:
  x4/1 -> Gain/1
  Real-Imag to Complex/1 -> Out1/1
  Delay24/1 -> Complex to Real-Imag/1
  Add1/1 -> Real-Imag to Complex/2
  Add/1 -> Real-Imag to Complex/1
  Complex to Real-Imag/2 -> Add/2, Add1/1
  Complex to Real-Imag/1 -> Add/1, Add1/2
  Gain/1 -> Delay1/1
  Delay1/1 -> Data Type Conversion/1
  Data Type Conversion/1 -> Delay24/1

== system fft_overlap_tomori/FFT64_outMuxed/64pointFFTchan/FFT64/multByMinusJ ==
  x4 : Inport
  Complex to Real-Imag : ComplexToRealImag
  Real-Imag to Complex : RealImagToComplex
  Unary Minus1 : UnaryMinus
  Out1 : Outport
  wires:
  Complex to Real-Imag/1 -> Unary Minus1/1
  Complex to Real-Imag/2 -> Real-Imag to Complex/1
  x4/1 -> Complex to Real-Imag/1
  Real-Imag to Complex/1 -> Out1/1
  Unary Minus1/1 -> Real-Imag to Complex/2

== system fft_overlap_tomori/FFT64_outMuxed/64pointFFTchan/FFT64/multByMinusJ3 ==
  In1 : Inport
  Complex to Real-Imag : ComplexToRealImag
  Real-Imag to Complex : RealImagToComplex
  Unary Minus1 : UnaryMinus
  Out1 : Outport
  wires:
  Complex to Real-Imag/1 -> Unary Minus1/1
  Complex to Real-Imag/2 -> Real-Imag to Complex/1
  In1/1 -> Complex to Real-Imag/1
  Real-Imag to Complex/1 -> Out1/1
  Unary Minus1/1 -> Real-Imag to Complex/2

== system fft_overlap_tomori/16//32 and test junk/16/FFT16/FFT8/multByExp(-j*Pi//4) ==
  In1 : Inport
  Add : Sum  OutDataTypeStr=fixed  RndMeth=Round
  Add1 : Sum  Inputs=+-  OutDataTypeStr=fixed  RndMeth=Round
  Complex to Real-Imag : ComplexToRealImag
  Delay24 : Delay
  Gain : Gain  Gain=sqrt(2)/2  ParamDataTypeStr=fixed  OutDataTypeStr=fixed  RndMeth=Round
  Real-Imag to Complex : RealImagToComplex
  Out1 : Outport
  wires:
  Real-Imag to Complex/1 -> Out1/1
  Gain/1 -> Delay24/1
  Complex to Real-Imag/1 -> Add1/2, Add/1
  Complex to Real-Imag/2 -> Add1/1, Add/2
  Add/1 -> Real-Imag to Complex/1
  Add1/1 -> Real-Imag to Complex/2
  Delay24/1 -> Complex to Real-Imag/1
  In1/1 -> Gain/1

== system fft_overlap_tomori/16//32 and test junk/16/FFT16/FFT8/multByExp(-j*Pi//4)1 ==
  In1 : Inport
  Add : Sum  OutDataTypeStr=fixed  RndMeth=Round
  Add1 : Sum  Inputs=+-  OutDataTypeStr=fixed  RndMeth=Round
  Complex to Real-Imag : ComplexToRealImag
  Delay24 : Delay
  Gain : Gain  Gain=sqrt(2)/2  ParamDataTypeStr=fixed  OutDataTypeStr=fixed  RndMeth=Round
  Real-Imag to Complex : RealImagToComplex
  Out1 : Outport
  wires:
  Real-Imag to Complex/1 -> Out1/1
  Gain/1 -> Delay24/1
  Complex to Real-Imag/1 -> Add1/2, Add/1
  Complex to Real-Imag/2 -> Add1/1, Add/2
  Add/1 -> Real-Imag to Complex/1
  Add1/1 -> Real-Imag to Complex/2
  Delay24/1 -> Complex to Real-Imag/1
  In1/1 -> Gain/1

== system fft_overlap_tomori/16//32 and test junk/16/FFT16/FFT8/multByMinusJ ==
  In1 : Inport
  Complex to Real-Imag : ComplexToRealImag
  Real-Imag to Complex : RealImagToComplex
  Unary Minus1 : UnaryMinus
  Out1 : Outport
  wires:
  Complex to Real-Imag/1 -> Unary Minus1/1
  Complex to Real-Imag/2 -> Real-Imag to Complex/1
  In1/1 -> Complex to Real-Imag/1
  Real-Imag to Complex/1 -> Out1/1
  Unary Minus1/1 -> Real-Imag to Complex/2

== system fft_overlap_tomori/16//32 and test junk/16/FFT16/FFT8/multByMinusJ1 ==
  In1 : Inport
  Complex to Real-Imag : ComplexToRealImag
  Real-Imag to Complex : RealImagToComplex
  Unary Minus1 : UnaryMinus
  Out1 : Outport
  wires:
  Unary Minus1/1 -> Real-Imag to Complex/2
  Real-Imag to Complex/1 -> Out1/1
  In1/1 -> Complex to Real-Imag/1
  Complex to Real-Imag/2 -> Real-Imag to Complex/1
  Complex to Real-Imag/1 -> Unary Minus1/1

== system fft_overlap_tomori/16//32 and test junk/16/FFT16/FFT8/multByMinusJ2 ==
  In1 : Inport
  Complex to Real-Imag : ComplexToRealImag
  Real-Imag to Complex : RealImagToComplex
  Unary Minus1 : UnaryMinus
  Out1 : Outport
  wires:
  Unary Minus1/1 -> Real-Imag to Complex/2
  Real-Imag to Complex/1 -> Out1/1
  In1/1 -> Complex to Real-Imag/1
  Complex to Real-Imag/2 -> Real-Imag to Complex/1
  Complex to Real-Imag/1 -> Unary Minus1/1

== system fft_overlap_tomori/16//32 and test junk/16/FFT16/FFT8/multByMinusJ3 ==
  In1 : Inport
  Complex to Real-Imag : ComplexToRealImag
  Real-Imag to Complex : RealImagToComplex
  Unary Minus1 : UnaryMinus
  Out1 : Outport
  wires:
  Complex to Real-Imag/1 -> Unary Minus1/1
  Complex to Real-Imag/2 -> Real-Imag to Complex/1
  In1/1 -> Complex to Real-Imag/1
  Real-Imag to Complex/1 -> Out1/1
  Unary Minus1/1 -> Real-Imag to Complex/2

== system fft_overlap_tomori/16//32 and test junk/16/FFT16/FFT8_1/multByExp(-j*Pi//4) ==
  In1 : Inport
  Add : Sum  OutDataTypeStr=fixed  RndMeth=Round
  Add1 : Sum  Inputs=+-  OutDataTypeStr=fixed  RndMeth=Round
  Complex to Real-Imag : ComplexToRealImag
  Delay24 : Delay
  Gain : Gain  Gain=sqrt(2)/2  ParamDataTypeStr=fixed  OutDataTypeStr=fixed  RndMeth=Round
  Real-Imag to Complex : RealImagToComplex
  Out1 : Outport
  wires:
  Real-Imag to Complex/1 -> Out1/1
  Gain/1 -> Delay24/1
  Complex to Real-Imag/1 -> Add1/2, Add/1
  Complex to Real-Imag/2 -> Add1/1, Add/2
  Add/1 -> Real-Imag to Complex/1
  Add1/1 -> Real-Imag to Complex/2
  Delay24/1 -> Complex to Real-Imag/1
  In1/1 -> Gain/1

== system fft_overlap_tomori/16//32 and test junk/16/FFT16/FFT8_1/multByExp(-j*Pi//4)1 ==
  In1 : Inport
  Add : Sum  OutDataTypeStr=fixed  RndMeth=Round
  Add1 : Sum  Inputs=+-  OutDataTypeStr=fixed  RndMeth=Round
  Complex to Real-Imag : ComplexToRealImag
  Delay24 : Delay
  Gain : Gain  Gain=sqrt(2)/2  ParamDataTypeStr=fixed  OutDataTypeStr=fixed  RndMeth=Round
  Real-Imag to Complex : RealImagToComplex
  Out1 : Outport
  wires:
  Real-Imag to Complex/1 -> Out1/1
  Gain/1 -> Delay24/1
  Complex to Real-Imag/1 -> Add1/2, Add/1
  Complex to Real-Imag/2 -> Add1/1, Add/2
  Add/1 -> Real-Imag to Complex/1
  Add1/1 -> Real-Imag to Complex/2
  Delay24/1 -> Complex to Real-Imag/1
  In1/1 -> Gain/1

== system fft_overlap_tomori/16//32 and test junk/16/FFT16/FFT8_1/multByMinusJ ==
  In1 : Inport
  Complex to Real-Imag : ComplexToRealImag
  Real-Imag to Complex : RealImagToComplex
  Unary Minus1 : UnaryMinus
  Out1 : Outport
  wires:
  Complex to Real-Imag/1 -> Unary Minus1/1
  Complex to Real-Imag/2 -> Real-Imag to Complex/1
  In1/1 -> Complex to Real-Imag/1
  Real-Imag to Complex/1 -> Out1/1
  Unary Minus1/1 -> Real-Imag to Complex/2

== system fft_overlap_tomori/16//32 and test junk/16/FFT16/FFT8_1/multByMinusJ1 ==
  In1 : Inport
  Complex to Real-Imag : ComplexToRealImag
  Real-Imag to Complex : RealImagToComplex
  Unary Minus1 : UnaryMinus
  Out1 : Outport
  wires:
  Unary Minus1/1 -> Real-Imag to Complex/2
  Real-Imag to Complex/1 -> Out1/1
  In1/1 -> Complex to Real-Imag/1
  Complex to Real-Imag/2 -> Real-Imag to Complex/1
  Complex to Real-Imag/1 -> Unary Minus1/1

== system fft_overlap_tomori/16//32 and test junk/16/FFT16/FFT8_1/multByMinusJ2 ==
  In1 : Inport
  Complex to Real-Imag : ComplexToRealImag
  Real-Imag to Complex : RealImagToComplex
  Unary Minus1 : UnaryMinus
  Out1 : Outport
  wires:
  Unary Minus1/1 -> Real-Imag to Complex/2
  Real-Imag to Complex/1 -> Out1/1
  In1/1 -> Complex to Real-Imag/1
  Complex to Real-Imag/2 -> Real-Imag to Complex/1
  Complex to Real-Imag/1 -> Unary Minus1/1

== system fft_overlap_tomori/16//32 and test junk/16/FFT16/FFT8_1/multByMinusJ3 ==
  In1 : Inport
  Complex to Real-Imag : ComplexToRealImag
  Real-Imag to Complex : RealImagToComplex
  Unary Minus1 : UnaryMinus
  Out1 : Outport
  wires:
  Complex to Real-Imag/1 -> Unary Minus1/1
  Complex to Real-Imag/2 -> Real-Imag to Complex/1
  In1/1 -> Complex to Real-Imag/1
  Real-Imag to Complex/1 -> Out1/1
  Unary Minus1/1 -> Real-Imag to Complex/2

== system fft_overlap_tomori/16//32 and test junk/16pointfftchan1/fft_res/cmut1/complexmult ==
  In1 : Inport
  In3 : Inport  Port=2
  Add1 : Sum  OutDataTypeStr=fixed_point  AccumDataTypeStr=fixed_point
  Add2 : Sum  OutDataTypeStr=fixed_point  AccumDataTypeStr=fixed_point
  Add3 : Sum  Inputs=+--  OutDataTypeStr=fixed_point  AccumDataTypeStr=fixed_point
  Add4 : Sum  Inputs=+-  OutDataTypeStr=fixed_point  AccumDataTypeStr=fixed_point
  Complex to Real-Imag : ComplexToRealImag
  Complex to Real-Imag1 : ComplexToRealImag
  Delay : Delay  DelayLength=3
  Delay1 : Delay  DelayLength=3
  Delay2 : Delay  DelayLength=3
  Product : Product  OutDataTypeStr=fixed_point
  Product1 : Product  OutDataTypeStr=fixed_point
  Product2 : Product  OutDataTypeStr=fixed_point
  Real-Imag to Complex : RealImagToComplex
  Out1 : Outport
  wires:
  Complex to Real-Imag1/2 -> Add1/2, Product2/2
  Complex to Real-Imag/2 -> Add2/2, Product2/1
  Complex to Real-Imag1/1 -> Add1/1, Product1/2
  Complex to Real-Imag/1 -> Add2/1, Product1/1
  Add1/1 -> Product/2
  Add2/1 -> Product/1
  Add3/1 -> Real-Imag to Complex/2
  Add4/1 -> Real-Imag to Complex/1
  Delay2/1 -> Add4/2, Add3/3
  Delay1/1 -> Add3/2, Add4/1
  Delay/1 -> Add3/1
  Real-Imag to Complex/1 -> Out1/1
  Product2/1 -> Delay2/1
  Product1/1 -> Delay1/1
  Product/1 -> Delay/1
  In3/1 -> Complex to Real-Imag1/1
  In1/1 -> Complex to Real-Imag/1

== system fft_overlap_tomori/16//32 and test junk/16pointfftchan1/fft_res/cmut2/complexmult ==
  In1 : Inport
  In3 : Inport  Port=2
  Add1 : Sum  OutDataTypeStr=fixed_point  AccumDataTypeStr=fixed_point
  Add2 : Sum  OutDataTypeStr=fixed_point  AccumDataTypeStr=fixed_point
  Add3 : Sum  Inputs=+--  OutDataTypeStr=fixed_point  AccumDataTypeStr=fixed_point
  Add4 : Sum  Inputs=+-  OutDataTypeStr=fixed_point  AccumDataTypeStr=fixed_point
  Complex to Real-Imag : ComplexToRealImag
  Complex to Real-Imag1 : ComplexToRealImag
  Delay : Delay  DelayLength=3
  Delay1 : Delay  DelayLength=3
  Delay2 : Delay  DelayLength=3
  Product : Product  OutDataTypeStr=fixed_point
  Product1 : Product  OutDataTypeStr=fixed_point
  Product2 : Product  OutDataTypeStr=fixed_point
  Real-Imag to Complex : RealImagToComplex
  Out1 : Outport
  wires:
  Complex to Real-Imag1/2 -> Add1/2, Product2/2
  Complex to Real-Imag/2 -> Add2/2, Product2/1
  Complex to Real-Imag1/1 -> Add1/1, Product1/2
  Complex to Real-Imag/1 -> Add2/1, Product1/1
  Add1/1 -> Product/2
  Add2/1 -> Product/1
  Add3/1 -> Real-Imag to Complex/2
  Add4/1 -> Real-Imag to Complex/1
  Delay2/1 -> Add4/2, Add3/3
  Delay1/1 -> Add3/2, Add4/1
  Delay/1 -> Add3/1
  Real-Imag to Complex/1 -> Out1/1
  Product2/1 -> Delay2/1
  Product1/1 -> Delay1/1
  Product/1 -> Delay/1
  In3/1 -> Complex to Real-Imag1/1
  In1/1 -> Complex to Real-Imag/1

== system fft_overlap_tomori/16//32 and test junk/16pointfftchan1/fft_res/cmut21/complexmult ==
  In1 : Inport
  In3 : Inport  Port=2
  Add1 : Sum  OutDataTypeStr=fixed_point  AccumDataTypeStr=fixed_point
  Add2 : Sum  OutDataTypeStr=fixed_point  AccumDataTypeStr=fixed_point
  Add3 : Sum  Inputs=+--  OutDataTypeStr=fixed_point  AccumDataTypeStr=fixed_point
  Add4 : Sum  Inputs=+-  OutDataTypeStr=fixed_point  AccumDataTypeStr=fixed_point
  Complex to Real-Imag : ComplexToRealImag
  Complex to Real-Imag1 : ComplexToRealImag
  Delay : Delay  DelayLength=3
  Delay1 : Delay  DelayLength=3
  Delay2 : Delay  DelayLength=3
  Product : Product  OutDataTypeStr=fixed_point
  Product1 : Product  OutDataTypeStr=fixed_point
  Product2 : Product  OutDataTypeStr=fixed_point
  Real-Imag to Complex : RealImagToComplex
  Out1 : Outport
  wires:
  Complex to Real-Imag1/2 -> Add1/2, Product2/2
  Complex to Real-Imag/2 -> Add2/2, Product2/1
  Complex to Real-Imag1/1 -> Add1/1, Product1/2
  Complex to Real-Imag/1 -> Add2/1, Product1/1
  Add1/1 -> Product/2
  Add2/1 -> Product/1
  Add3/1 -> Real-Imag to Complex/2
  Add4/1 -> Real-Imag to Complex/1
  Delay2/1 -> Add4/2, Add3/3
  Delay1/1 -> Add3/2, Add4/1
  Delay/1 -> Add3/1
  Real-Imag to Complex/1 -> Out1/1
  Product2/1 -> Delay2/1
  Product1/1 -> Delay1/1
  Product/1 -> Delay/1
  In3/1 -> Complex to Real-Imag1/1
  In1/1 -> Complex to Real-Imag/1

== system fft_overlap_tomori/16//32 and test junk/16pointfftchan1/fft_res/cmut3/complexmult ==
  In1 : Inport
  In3 : Inport  Port=2
  Add1 : Sum  OutDataTypeStr=fixed_point  AccumDataTypeStr=fixed_point
  Add2 : Sum  OutDataTypeStr=fixed_point  AccumDataTypeStr=fixed_point
  Add3 : Sum  Inputs=+--  OutDataTypeStr=fixed_point  AccumDataTypeStr=fixed_point
  Add4 : Sum  Inputs=+-  OutDataTypeStr=fixed_point  AccumDataTypeStr=fixed_point
  Complex to Real-Imag : ComplexToRealImag
  Complex to Real-Imag1 : ComplexToRealImag
  Delay : Delay  DelayLength=3
  Delay1 : Delay  DelayLength=3
  Delay2 : Delay  DelayLength=3
  Product : Product  OutDataTypeStr=fixed_point
  Product1 : Product  OutDataTypeStr=fixed_point
  Product2 : Product  OutDataTypeStr=fixed_point
  Real-Imag to Complex : RealImagToComplex
  Out1 : Outport
  wires:
  Complex to Real-Imag1/2 -> Add1/2, Product2/2
  Complex to Real-Imag/2 -> Add2/2, Product2/1
  Complex to Real-Imag1/1 -> Add1/1, Product1/2
  Complex to Real-Imag/1 -> Add2/1, Product1/1
  Add1/1 -> Product/2
  Add2/1 -> Product/1
  Add3/1 -> Real-Imag to Complex/2
  Add4/1 -> Real-Imag to Complex/1
  Delay2/1 -> Add4/2, Add3/3
  Delay1/1 -> Add3/2, Add4/1
  Delay/1 -> Add3/1
  Real-Imag to Complex/1 -> Out1/1
  Product2/1 -> Delay2/1
  Product1/1 -> Delay1/1
  Product/1 -> Delay/1
  In3/1 -> Complex to Real-Imag1/1
  In1/1 -> Complex to Real-Imag/1

== system fft_overlap_tomori/16//32 and test junk/16pointfftchan1/fft_res/fft_1/proddd ==
  In1 : Inport
  Delay24 : Delay  DelayLength=1
  Gain : Gain  Gain=fi(sqrt(2)/2,1,16,15)  ParamDataTypeStr=fixdt(1,16,15)  OutDataTypeStr=fixed_point
  s3 : Subsystem
  Out1 : Outport
  wires:
  Delay24/1 -> s3/1(In1)
  Gain/1 -> Delay24/1
  In1/1 -> Gain/1
  s3/1(Out1) -> Out1/1

== system fft_overlap_tomori/16//32 and test junk/16pointfftchan1/fft_res/fft_1/ptrrt ==
  In1 : Inport
  Delay25 : Delay  DelayLength=1
  Gain1 : Gain  Gain=fi(-sqrt(2)/2,1,16,15)  ParamDataTypeStr=fixdt(1,16,15)  OutDataTypeStr=fixed_point
  s4 : Subsystem
  Out1 : Outport
  wires:
  Gain1/1 -> Delay25/1
  Delay25/1 -> s4/1(In1)
  In1/1 -> Gain1/1
  s4/1(Out1) -> Out1/1

== system fft_overlap_tomori/16//32 and test junk/16pointfftchan1/fft_res/fft_1/s1 ==
  In1 : Inport
  Complex to Real-Imag : ComplexToRealImag
  Real-Imag to Complex : RealImagToComplex
  Unary Minus : UnaryMinus
  Out1 : Outport  VectorParamsAs1DForOutWhenUnconnected=off
  wires:
  Real-Imag to Complex/1 -> Out1/1
  Unary Minus/1 -> Real-Imag to Complex/2
  Complex to Real-Imag/1 -> Unary Minus/1
  Complex to Real-Imag/2 -> Real-Imag to Complex/1
  In1/1 -> Complex to Real-Imag/1

== system fft_overlap_tomori/16//32 and test junk/16pointfftchan1/fft_res/fft_1/s17 ==
  In1 : Inport
  Complex to Real-Imag : ComplexToRealImag
  Real-Imag to Complex : RealImagToComplex
  Unary Minus : UnaryMinus
  Out1 : Outport  VectorParamsAs1DForOutWhenUnconnected=off
  wires:
  In1/1 -> Complex to Real-Imag/1
  Complex to Real-Imag/2 -> Real-Imag to Complex/1
  Complex to Real-Imag/1 -> Unary Minus/1
  Unary Minus/1 -> Real-Imag to Complex/2
  Real-Imag to Complex/1 -> Out1/1

== system fft_overlap_tomori/16//32 and test junk/16pointfftchan1/fft_res/fft_1/s2 ==
  In1 : Inport
  Complex to Real-Imag : ComplexToRealImag
  Real-Imag to Complex : RealImagToComplex
  Unary Minus : UnaryMinus
  Out1 : Outport  VectorParamsAs1DForOutWhenUnconnected=off
  wires:
  Real-Imag to Complex/1 -> Out1/1
  Unary Minus/1 -> Real-Imag to Complex/2
  Complex to Real-Imag/1 -> Unary Minus/1
  Complex to Real-Imag/2 -> Real-Imag to Complex/1
  In1/1 -> Complex to Real-Imag/1

== system fft_overlap_tomori/16//32 and test junk/16pointfftchan1/fft_res/fft_8/proddd ==
  In1 : Inport
  Delay24 : Delay  DelayLength=1
  Gain : Gain  Gain=fi(sqrt(2)/2,1,16,15)  ParamDataTypeStr=fixdt(1,16,15)  OutDataTypeStr=fixed_point
  s3 : Subsystem
  Out1 : Outport
  wires:
  s3/1(Out1) -> Out1/1
  In1/1 -> Gain/1
  Gain/1 -> Delay24/1
  Delay24/1 -> s3/1(In1)

== system fft_overlap_tomori/16//32 and test junk/16pointfftchan1/fft_res/fft_8/ptrrt ==
  In1 : Inport
  Delay25 : Delay  DelayLength=1
  Gain1 : Gain  Gain=fi(-sqrt(2)/2,1,16,15)  ParamDataTypeStr=fixdt(1,16,15)  OutDataTypeStr=fixed_point
  s4 : Subsystem
  Out1 : Outport
  wires:
  s4/1(Out1) -> Out1/1
  In1/1 -> Gain1/1
  Delay25/1 -> s4/1(In1)
  Gain1/1 -> Delay25/1

== system fft_overlap_tomori/16//32 and test junk/16pointfftchan1/fft_res/fft_8/s1 ==
  In1 : Inport
  Complex to Real-Imag : ComplexToRealImag
  Real-Imag to Complex : RealImagToComplex
  Unary Minus : UnaryMinus
  Out1 : Outport  VectorParamsAs1DForOutWhenUnconnected=off
  wires:
  In1/1 -> Complex to Real-Imag/1
  Complex to Real-Imag/2 -> Real-Imag to Complex/1
  Complex to Real-Imag/1 -> Unary Minus/1
  Unary Minus/1 -> Real-Imag to Complex/2
  Real-Imag to Complex/1 -> Out1/1

== system fft_overlap_tomori/16//32 and test junk/16pointfftchan1/fft_res/fft_8/s17 ==
  In1 : Inport
  Complex to Real-Imag : ComplexToRealImag
  Real-Imag to Complex : RealImagToComplex
  Unary Minus : UnaryMinus
  Out1 : Outport  VectorParamsAs1DForOutWhenUnconnected=off
  wires:
  Real-Imag to Complex/1 -> Out1/1
  Unary Minus/1 -> Real-Imag to Complex/2
  Complex to Real-Imag/1 -> Unary Minus/1
  Complex to Real-Imag/2 -> Real-Imag to Complex/1
  In1/1 -> Complex to Real-Imag/1

== system fft_overlap_tomori/16//32 and test junk/16pointfftchan1/fft_res/fft_8/s2 ==
  In1 : Inport
  Complex to Real-Imag : ComplexToRealImag
  Real-Imag to Complex : RealImagToComplex
  Unary Minus : UnaryMinus
  Out1 : Outport  VectorParamsAs1DForOutWhenUnconnected=off
  wires:
  In1/1 -> Complex to Real-Imag/1
  Complex to Real-Imag/2 -> Real-Imag to Complex/1
  Complex to Real-Imag/1 -> Unary Minus/1
  Unary Minus/1 -> Real-Imag to Complex/2
  Real-Imag to Complex/1 -> Out1/1

== system fft_overlap_tomori/16//32 and test junk/16pointfftchan1/fft_res/prod_2/s3 ==
  In1 : Inport
  Add16 : Sum  OutDataTypeStr=fixed_point  AccumDataTypeStr=fixed_point
  Add21 : Sum  Inputs=+-  OutDataTypeStr=fixed_point  AccumDataTypeStr=fixed_point
  Complex to Real-Imag : ComplexToRealImag
  Real-Imag to Complex : RealImagToComplex
  Out1 : Outport  VectorParamsAs1DForOutWhenUnconnected=off
  wires:
  Add21/1 -> Real-Imag to Complex/2
  Add16/1 -> Real-Imag to Complex/1
  Complex to Real-Imag/2 -> Add16/2, Add21/1
  Complex to Real-Imag/1 -> Add16/1, Add21/2
  In1/1 -> Complex to Real-Imag/1
  Real-Imag to Complex/1 -> Out1/1

== system fft_overlap_tomori/16//32 and test junk/16pointfftchan1/fft_res/prod_3/s4 ==
  In1 : Inport
  Add16 : Sum  OutDataTypeStr=fixed_point  AccumDataTypeStr=fixed_point
  Add21 : Sum  Inputs=+-  OutDataTypeStr=fixed_point  AccumDataTypeStr=fixed_point
  Complex to Real-Imag : ComplexToRealImag
  Real-Imag to Complex : RealImagToComplex
  Out1 : Outport  VectorParamsAs1DForOutWhenUnconnected=off
  wires:
  Add16/1 -> Real-Imag to Complex/2
  Add21/1 -> Real-Imag to Complex/1
  Complex to Real-Imag/2 -> Add21/2, Add16/2
  Complex to Real-Imag/1 -> Add21/1, Add16/1
  Real-Imag to Complex/1 -> Out1/1
  In1/1 -> Complex to Real-Imag/1
